simulink model "test1"  (R2017b)
settings: Solver=VariableStepAuto  StartTime=0.0  StopTime=T_stop  RelTol=1e-3
values from neighbouring files (symbols this model uses):
  da = 0    [AC_L15_Example1.m]    (also in AC_L15_Example2.m = 1; AC_L16_1.m = 1; AC_L16_2.m)
  dy = 0    [AC_L15_Example1.m]    (also in AC_L15_Example2.m; AC_L16_1.m; AC_L16_2.m)
  r_s = -1    [AC_L15_Example1.m]    (also in AC_L15_Example2.m = 1; AC_L16_2.m)
  rho = 0    [AC_L15_Example2.m]    (also in AC_L16_1.m)
libraries: cstblocks x2, simulink x2
settings Model: Creator=hantao.li  LastModifiedBy=hantao.li

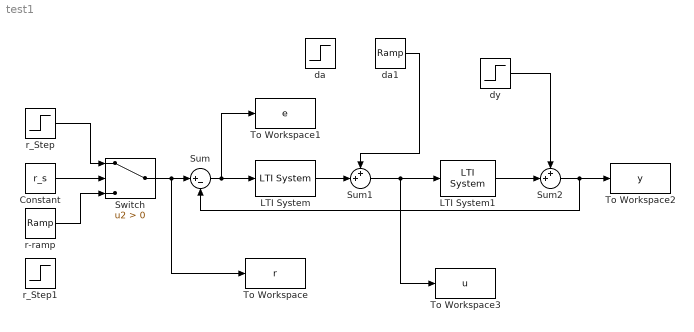
== system test1 ==
  Constant : Constant  Value=r_s
  LTI System : cstblocks/LTI System  sys=C  IC=[]
  LTI System1 : cstblocks/LTI System  sys=G  IC=[]
  Sum : Sum  Inputs=|+-
  Sum1 : Sum  Inputs=++|
  Sum2 : Sum  Inputs=++|
  Switch : Switch  Criteria=u2 > Threshold
  To Workspace : ToWorkspace  VariableName=r  SaveFormat=Timeseries  SampleTime=-1
  To Workspace1 : ToWorkspace  VariableName=e  SaveFormat=Timeseries  SampleTime=-1
  To Workspace2 : ToWorkspace  VariableName=y  SaveFormat=Timeseries  SampleTime=-1
  To Workspace3 : ToWorkspace  VariableName=u  SaveFormat=Timeseries  SampleTime=-1
  da : Step  Time=0  After=da  SampleTime=0
  da1 : simulink/Sources/Ramp  slope=da  start=0  X0=0
  dy : Step  Time=0  After=dy  SampleTime=0
  r-ramp : simulink/Sources/Ramp  slope=rho  start=0  X0=0
  r_Step : Step  Time=0  SampleTime=0
  r_Step1 : Step  Time=0  After=rho  SampleTime=0
  wires:
  r_Step/1 -> Switch/1
  Sum/1 -> To Workspace1/1, LTI System/1
  Switch/1 -> To Workspace/1, Sum/1
  Sum1/1 -> To Workspace3/1, LTI System1/1
  LTI System/1 -> Sum1/2
  Sum2/1 -> Sum/2, To Workspace2/1
  LTI System1/1 -> Sum2/2
  dy/1 -> Sum2/1
  Constant/1 -> Switch/2
  da1/1 -> Sum1/1
  r-ramp/1 -> Switch/3
